simulink model "TankFilling2"  (R2020b)
settings: Solver=VariableStepAuto  StartTime=0.0  StopTime=5000  RelTol=1e-3
values from neighbouring files (symbols this model uses):
  a_in = 1    [TankFillingScript.m]
  a_out = 0    [TankFillingScript.m]
  c = 16    [TankFillingScript.m]
  Q_in = 1    [TankFillingScript.m]
undefined symbols (not defined in the file or in its folder): l_out
settings Model: Creator=StevensUser  LastModifiedBy=mreiff

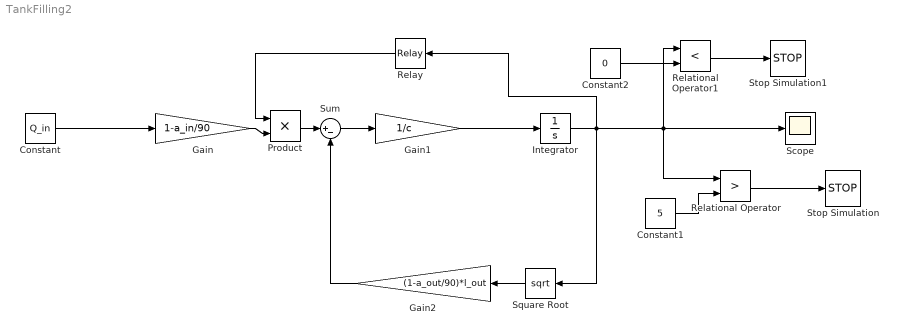
== system TankFilling2 ==
  Constant : Constant  Value=Q_in
  Constant1 : Constant  Value=5
  Constant2 : Constant  Value=0
  Gain : Gain  Gain=1-a_in/90
  Gain1 : Gain  Gain=1/c
  Gain2 : Gain  Gain=(1-a_out/90)*l_out
  Integrator : Integrator
  Product : Product
  Relational Operator : RelationalOperator  Operator=>  OutDataTypeStr=boolean  RndMeth=Simplest
  Relational Operator1 : RelationalOperator  Operator=<  OutDataTypeStr=boolean  RndMeth=Simplest
  Relay : Relay  OnSwitchValue=4.1  OffSwitchValue=3.9  OnOutputValue=0  OffOutputValue=1
  Scope : Scope
  Square Root : Sqrt  SaturateOnIntegerOverflow=on
  Stop Simulation : Stop
  Stop Simulation1 : Stop
  Sum : Sum  Inputs=|+-
  wires:
  Constant/1 -> Gain/1
  Gain1/1 -> Integrator/1
  Relational Operator/1 -> Stop Simulation/1
  Constant1/1 -> Relational Operator/2
  Sum/1 -> Gain1/1
  Gain2/1 -> Sum/2
  Square Root/1 -> Gain2/1
  Constant2/1 -> Relational Operator1/2
  Relational Operator1/1 -> Stop Simulation1/1
  Gain/1 -> Product/2
  Product/1 -> Sum/1
  Integrator/1 -> Square Root/1, Relational Operator/1, Scope/1, Relational Operator1/1, Relay/1
  Relay/1 -> Product/1
